simulink model "ES247A_MotAgCmp"  (R2013b)
settings: Solver=VariableStepDiscrete  SolverMode=SingleTasking  StartTime=0.0  StopTime=1  FixedStep=0.002  RelTol=1e-3
values from neighbouring files (symbols this model uses):
  MOTAGCMPENAMASK_CNT_U08 = DataDict.Constant    [ES247A_MotAgCmp_DataDict.m]
  MOTAGCMPMECLDEGPERREV_DEGPERREV_U16P0 = DataDict.Constant    [ES247A_MotAgCmp_DataDict.m]
  MOTAGCUMVALGNDMASK_CNT_U32 = DataDict.Constant    [ES247A_MotAgCmp_DataDict.m]
  MOTAGCUMVALGNDMRFREVMASK_CNT_U32 = DataDict.Constant    [ES247A_MotAgCmp_DataDict.m]
  MOTAGDELTALIM_MOTREV_U0P16 = DataDict.Constant    [ES247A_MotAgCmp_DataDict.m]
  MOTAGMAXDELTA_MOTREV_U0P16 = DataDict.Constant    [ES247A_MotAgCmp_DataDict.m]
  SysGlbPrmMotPoleCnt = DataDict.ImprtdCal    [ES247A_MotAgCmp_DataDict.m]
  SysGlbPrmSysKineRat = DataDict.ImprtdCal    [ES247A_MotAgCmp_DataDict.m]
undefined symbols (not defined in the file or in its folder): sigbuilder_block
libraries: simulink x8, NexteerUtilities x4, FixdToFloat x1
(part 1 of 2)
settings Model: Creator=pz79n7  LastModifiedBy=tzbsjd
settings SolverCC: AutoInsertRateTranBlk=on  InsertRTBMode=Always
settings DataIOCC: LimitDataPoints=off  SaveFormat=Structure  ReturnWorkspaceOutputs=on
settings OptimizationCC: BlockReduction=off  InlineParams=on  ZeroExternalMemoryAtStartup=off  ZeroInternalMemoryAtStartup=off  OptimizeModelRefInitCode=on  LifeSpan=1
settings DebuggingCC: SignalInfNanChecking=error  SignalRangeChecking=warning  UnderspecifiedInitializationDetection=Simplified  SolverPrmCheckMsg=error  InheritedTsInSrcMsg=error  DiscreteInheritContinuousMsg=error  SingleTaskRateTransMsg=error  TasksWithSamePriorityMsg=error  SigSpecEnsureSampleTimeMsg=error  CheckMatrixSingularityMsg=error  ParameterUnderflowMsg=error  ParameterPrecisionLossMsg=error  ParameterTunabilityLossMsg=error  FixptConstUnderflowMsg=warning  FixptConstOverflowMsg=warning  VectorMatrixConversionMsg=error  SignalLabelMismatchMsg=error  UnconnectedInputMsg=error  UnconnectedOutputMsg=error  UnconnectedLineMsg=error  SFcnCompatibilityMsg=error  UniqueDataStoreMsg=warning  BusObjectLabelMismatch=error  RootOutportRequireBusObject=error  AssertControl=DisableAll  ModelReferenceIOMsg=error  ModelReferenceVersionMismatchMessage=warning  ModelReferenceIOMismatchMessage=error  ModelReferenceCSMismatchMessage=warning  ModelReferenceDataLoggingMessage=error  StateNameClashWarn=warning  StrictBusMsg=ErrorOnBusTreatedAsVector  NonBusSignalsTreatedAsBus=error  SFUnexpectedBacktrackingDiag=error  SFInvalidInputDataAccessInChartInitDiag=error  SFNoUnconditionalDefaultTransitionDiag=error  SFTransitionOutsideNaturalParentDiag=error  SFUnconditionalTransitionShadowingDiag=error  SFUndirectedBroadcastEventsDiag=error
settings ModelReferenceCC: ModelReferenceNumInstancesAllowed=Single
settings RTWCC: SystemTargetFile=autosar.tlc  GenCodeOnly=on  TemplateMakefile=ert_default_tmf  Description=AUTOSAR  GenerateReport=on  ProcessScript=autosar_make_rtw_hook  LaunchReport=on
settings CodeAppCC: GenerateComments=off  IgnoreCustomStorageClasses=off  CustomSymbolStrType=$N$R$M  CustomSymbolStrBlkIO=$N$M  SimulinkBlockComments=off
settings STFCustomTargetCC: ParMdlRefBuildCompliant=on  CompOptLevelCompliant=on  IncludeMdlTerminateFcn=off  CombineOutputUpdateFcns=on  SuppressErrorStatus=on  ERTFirstTimeCompliant=on  ERTCustomFileBanners=on  SupportNonFinite=off  SupportComplex=off  SupportContinuousTime=off  SupportNonInlinedSFcns=off  MATLABClassNameForMDSCustomization=Simulink.SoftwareTarget.ERTCustomization  AutosarCompliant=on  GRTInterface=off  SystemTargetFile=autosar.tlc
settings ERTTargetCC: CodeReplacementLibrary=ANSI_C  ConcurrentExecutionCompliant=off  IncludeMdlTerminateFcn=off  SuppressErrorStatus=on  SupportNonFinite=off  SupportComplex=off  ModelStepFunctionPrototypeControlCompliant=off  CPPClassGenCompliant=off  AutosarCompliant=on  InlinedParameterPlacement=NonHierarchical  ERTCustomFileTemplate=example_file_process.tlc  EnableUserReplacementTypes=on

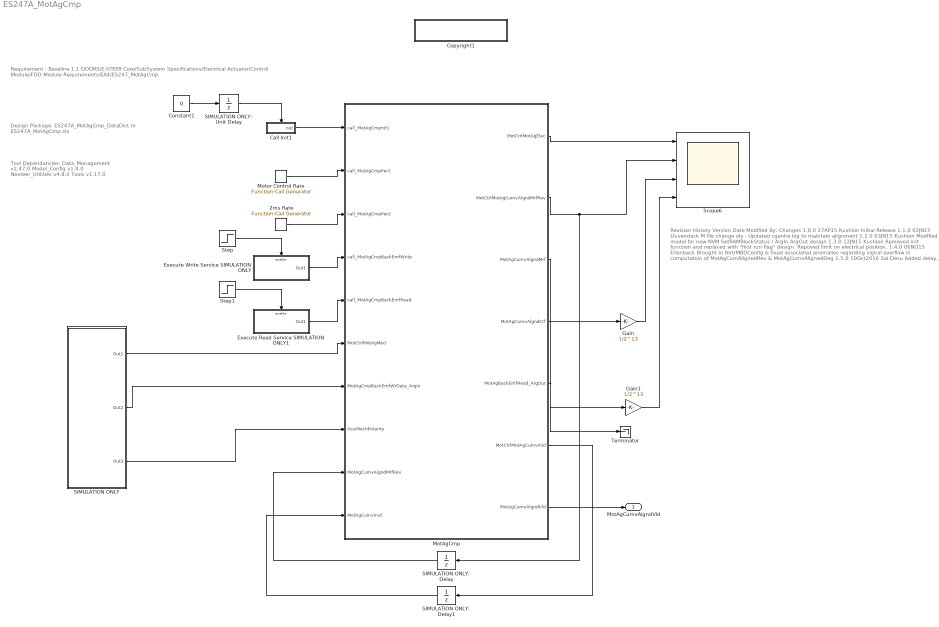
== system ES247A_MotAgCmp ==
  note: Revision History
      |
      | Version		Date 		Modified By: 		Changes
      | 1.0.0	 	27AP15		Kushion			Initial Release
      | 1.1.0		02JN15		Duvendack		M file change oly - Updated cganhe log to maintain alignment
      | 1.2.0		03JN15		Kushion			Modified model for new NVM SetRAMBlockStatus / ArgIn ArgOut design
      | 1.3.0		12JN15		Kushion			Removed init function and replaced with "first run flag" design.  Repoved limit on electrical position.
      | 1.4.0		06NO15		Erlenbeck		Brought in NxtrMBDConfig & fixed associated anomalies regarding signal overflow in computatoin
      | 										of MotAgCumAlignedRev & MotAgCumvAlignedDeg
      | 1.5.0              10Oct2016     Sai Desu              Added delay to use MotCntrlMotAgMecl
      | 1.6.0              19Oct2016     Sai Desu             Moved MotAgCmpMotCtrlMotAgMeclPrev store to outside of the subsystem
      | 1.7.0               11Nov2016    Sai Desu             Added a new PIM DigMotHwPosn for EMC Validation
  note: Tool Dependancies:
      | Data_Management v2.47.0
      | Model_Config v1.4.0
      | Nexteer_Utilities v4.8.0
      | Tools v1.17.0
  note: Requirement : Baseline 1.1
      | DOORS/E-STEER Core/SubSystem Specifications/Electrical Actuator/Control Module/FDD Module Requirements/EA4/ES247_MotAgCmp
  note: Design Package:
      | ES247A_MotAgCmp_DataDict.m
      | ES247A_MotAgCmp.slx
  2ms Rate : simulink/Ports & Subsystems/Function-Call Generator  sample_time=0.002  numberOfIterations=1
  Call Init1 : Subsystem  TreatAsAtomicUnit=on
  Constant1 : Constant  Value=0  OutDataTypeStr=uint8
  Copyright1 : Subsystem  Description=|  mask(Copyright Information){none=on}
      | Copyright info block.                                               
      |                                                                     
      | Place copyright information at the top of every subsystem in design.
      mask prompts: none "No parameters"
      mask help: Place copyright information at the top of every subsystem in design.
      mask Display:
      | NxtrConf = 'Nexteer Confidential';
      | 
      | sys = bdroot; %handle for the current model ("system")
      | first = get_param(sys,'Created');
      | if(isempty(first))
      |     first = datestr(now,'yyyy');
      | else
      |     first = first(end-3:end);  %year is last four digits
      | end
      | 
      | last = get_param(sys,'LastModifiedDate');
      | if isempty(last)
      |     last = datestr(now,'yyyy');
      | else
      |     last = last(end-3:end);
      | end
      | 
      | if strcmp(first,last)
      |     fprintf('%s\nCopyright  %s Nexteer',NxtrConf,first);
      | else
      |     fprintf('%s\n%s%s-%s Nexteer',NxtrConf,char(169),first,last);
      | end
  Execute Read Service SIMULATION ONLY1 : Subsystem  TreatAsAtomicUnit=on
  Execute Write Service SIMULATION ONLY : Subsystem  TreatAsAtomicUnit=on
  Gain : Gain  Gain=1/2^13
  Gain1 : Gain  Gain=1/2^13
  MotAgCmp : Subsystem
  Motor Control Rate : simulink/Ports & Subsystems/Function-Call Generator  sample_time=0.0000625  numberOfIterations=1
  SIMULATION ONLY : Subsystem
  SIMULATION ONLY: Delay : UnitDelay  SampleTime=-1
  SIMULATION ONLY: Delay1 : UnitDelay  SampleTime=-1
  SIMULATION ONLY: Unit Delay : UnitDelay  InitialCondition=1  SampleTime=-1
  Scope6 : Scope  NumInputPorts=4
      settings: YMin=0~-1e+08~-200000~-200000  YMax=70000~1.1e+09~200000~200000  SaveName=ScopeData5  MaxDataPoints=100000
  Step : Step  Time=4.175  SampleTime=0
  Step1 : Step  Time=4.185  SampleTime=0
  Terminator : Terminator
  MotAgCumvAlgndVld : Outport  RequirementInfo={} %GIDa_42b80226_dd05_44ce_a302_5ea1a8b1de89
  wires:
  MotAgCmp/1(MotCtrlMotAgElec) -> Scope6/1
  MotAgCmp/2(MotCtrlMotAgCumvAlgndMrfRev) -> SIMULATION ONLY: Delay/1, Scope6/2
  Motor Control Rate/1 -> MotAgCmp/2(call_MotAgCmpPer1)
  Execute Write Service SIMULATION ONLY/1(Out1) -> MotAgCmp/4(call_MotAgCmpBackEmfWrite)
  Step/1 -> Execute Write Service SIMULATION ONLY/Enable
  2ms Rate/1 -> MotAgCmp/3(call_MotAgCmpPer2)
  MotAgCmp/3(MotAgCumvAlgndMrf) -> Gain/1
  MotAgCmp/4(MotAgCumvAlgndCrf) -> Gain1/1
  SIMULATION ONLY/3(Out3) -> MotAgCmp/8(AssiMechPolarity)
  SIMULATION ONLY/1(Out1) -> MotAgCmp/6(MotCtrlMotAgMecl)
  SIMULATION ONLY/2(Out2) -> MotAgCmp/7(MotAgCmpBackEmfWrData_ArgIn)
  Execute Read Service SIMULATION ONLY1/1(Out1) -> MotAgCmp/5(call_MotAgCmpBackEmfRead)
  Step1/1 -> Execute Read Service SIMULATION ONLY1/Enable
  Gain/1 -> Scope6/3
  Gain1/1 -> Scope6/4
  MotAgCmp/5(MotAgBackEmfRead_ArgOut) -> Terminator/1
  SIMULATION ONLY: Delay/1 -> MotAgCmp/9(MotAgCumvAlgndMrfRev)
  MotAgCmp/6(MotCtrlMotAgCumvInid) -> SIMULATION ONLY: Delay1/1
  Constant1/1 -> SIMULATION ONLY: Unit Delay/1
  SIMULATION ONLY: Unit Delay/1 -> Call Init1/Enable
  Call Init1/1(out) -> MotAgCmp/1(call_MotAgCmpnit1)
  SIMULATION ONLY: Delay1/1 -> MotAgCmp/10(MotAgCumvInid)
  MotAgCmp/7(MotAgCumvAlgndVld) -> MotAgCumvAlgndVld/1

== system ES247A_MotAgCmp/Call Init1 ==
  Enable : EnablePort
  Function Call Trigger : simulink/Ports & Subsystems/Function-Call Generator  RequirementInfo={} %GIDa_a6a4a62e_0f67_4a31_8bd8_36e712ec7718  sample_time=0.002  numberOfIterations=1
  out : Outport
  wires:
  Function Call Trigger/1 -> out/1

== system ES247A_MotAgCmp/Copyright1 ==

== system ES247A_MotAgCmp/Execute Read Service SIMULATION ONLY1 ==
  Enable : EnablePort
  Function-Call Generator1 : simulink/Ports & Subsystems/Function-Call Generator  sample_time=0.0000625  numberOfIterations=1
  Out1 : Outport
  wires:
  Function-Call Generator1/1 -> Out1/1

== system ES247A_MotAgCmp/Execute Write Service SIMULATION ONLY ==
  Enable : EnablePort
  Function-Call Generator1 : simulink/Ports & Subsystems/Function-Call Generator  sample_time=0.0000625  numberOfIterations=1
  Out1 : Outport
  wires:
  Function-Call Generator1/1 -> Out1/1

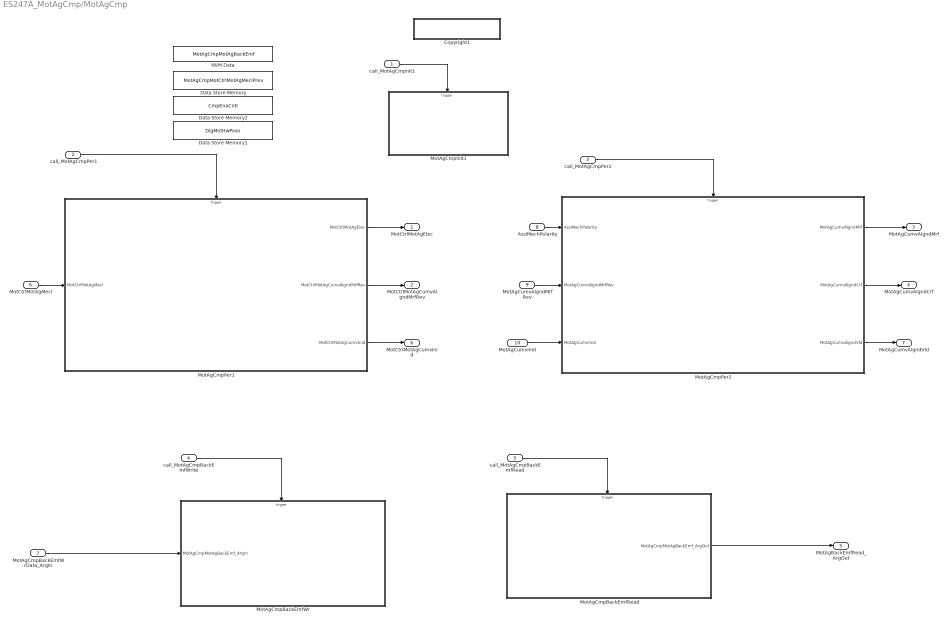
== system ES247A_MotAgCmp/MotAgCmp ==
  call_MotAgCmpnit1 : Inport  RequirementInfo={} %GIDa_7be01678_764c_45c5_827a_c2415c53d3c3
  call_MotAgCmpPer1 : Inport  RequirementInfo={'linktype_rmi_doors' '0000cf60 (/E-STEER Core/SubSystem Specifications/Electrical Actuator/Control Module/FDD Module Requirements/EA4/ES247A_MotAgCmp DRAFT)' '#ES247A_75' 'true' 'REQ: ES247A_75' '' } %GIDa_c4a7fd40_4a5d_4f59_ada5_16c56c4fb6c4  Port=2
  call_MotAgCmpPer2 : Inport  RequirementInfo={} %GIDa_2d6987ea_2640_46d5_a436_3696734fd2e8  Port=3
  call_MotAgCmpBackEmfWrite : Inport  Port=4
  call_MotAgCmpBackEmfRead : Inport  Port=5
  MotCtrlMotAgMecl : Inport  RequirementInfo={'linktype_rmi_doors' '0000cf60 (/E-STEER Core/SubSystem Specifications/Electrical Actuator/Control Module/FDD Module Requirements/EA4/ES247A_MotAgCmp DRAFT)' '#ES247A_48' 'true' 'REQ: ES247A_48' '' } %GIDa_c8a552f0_582e_4578_bd53_0d3cc336a1f5  Port=6
  MotAgCmpBackEmfWrData_ArgIn : Inport  Port=7
  AssiMechPolarity : Inport  RequirementInfo={'linktype_rmi_doors' '0000cf60 (/E-STEER Core/SubSystem Specifications/Electrical Actuator/Control Module/FDD Module Requirements/EA4/ES247A_MotAgCmp DRAFT)' '#ES247A_49' 'true' 'REQ: ES247A_49' '' } %GIDa_2804f92e_c79f_4452_aaac_51e06974467c  Port=8
  MotAgCumvAlgndMrfRev : Inport  RequirementInfo={'linktype_rmi_doors' '0000cf60 (/E-STEER Core/SubSystem Specifications/Electrical Actuator/Control Module/FDD Module Requirements/EA4/ES247A_MotAgCmp DRAFT)' '#ES247A_49' 'true' 'REQ: ES247A_49' '' } %GIDa_aef0170f_c17e_4400_b85e_a6e7f6d587e0  Port=9
  MotAgCumvInid : Inport  Port=10
  Copyright1 : Subsystem  Description=|  mask(Copyright Information){none=on}
      | Copyright info block.                                               
      |                                                                     
      | Place copyright information at the top of every subsystem in design.
      mask prompts: none "No parameters"
      mask help: Place copyright information at the top of every subsystem in design.
      mask Display:
      | NxtrConf = 'Nexteer Confidential';
      | 
      | sys = bdroot; %handle for the current model ("system")
      | first = get_param(sys,'Created');
      | if(isempty(first))
      |     first = datestr(now,'yyyy');
      | else
      |     first = first(end-3:end);  %year is last four digits
      | end
      | 
      | last = get_param(sys,'LastModifiedDate');
      | if isempty(last)
      |     last = datestr(now,'yyyy');
      | else
      |     last = last(end-3:end);
      | end
      | 
      | if strcmp(first,last)
      |     fprintf('%s\nCopyright  %s Nexteer',NxtrConf,first);
      | else
      |     fprintf('%s\n%s%s-%s Nexteer',NxtrConf,char(169),first,last);
      | end
  Data Store Memory : DataStoreMemory  DataStoreName=MotAgCmpMotCtrlMotAgMeclPrev  StateMustResolveToSignalObject=on
  Data Store Memory1 : DataStoreMemory  DataStoreName=DigMotHwPosn  OutDataTypeStr=single  StateMustResolveToSignalObject=on
  Data Store Memory2 : DataStoreMemory  DataStoreName=CmpEnaCntr  OutDataTypeStr=uint8  StateMustResolveToSignalObject=on
  MotAgCmpBackEmfRead : Subsystem  RequirementInfo={'linktype_rmi_doors' '0000cf60 (/E-STEER Core/SubSystem Specifications/Electrical Actuator/Control Module/FDD Module Requirements/EA4/ES247A_MotAgCmp DRAFT)' '#ES247A_71' 'true' 'REQ: ES247A_71' '' } %GIDa_3ab88c9c_8789_4b0d_9902_4656dd01c1af
  MotAgCmpBackEmfWr : Subsystem  RequirementInfo={'linktype_rmi_doors' '0000cf60 (/E-STEER Core/SubSystem Specifications/Electrical Actuator/Control Module/FDD Module Requirements/EA4/ES247A_MotAgCmp DRAFT)' '#ES247A_32' 'true' 'REQ: ES247A_32' '' } %GIDa_04a0761c_e8f1_4ec8_a62e_de9528ead8f5
  MotAgCmpInit1 : Subsystem
  MotAgCmpPer1 : Subsystem
  MotAgCmpPer2 : Subsystem  RequirementInfo={'linktype_rmi_doors' '0000cf60 (/E-STEER Core/SubSystem Specifications/Electrical Actuator/Control Module/FDD Module Requirements/EA4/ES247A_MotAgCmp DRAFT)' '#ES247A_81' 'true' 'REQ: ES247A_81' '' ; 'linktype_rmi_doors' '0000cf60 (/E-STEER Core/SubSystem Specifications/Electrical Actuator/Control Module/FDD Module Requirements/EA4/ES247A_MotAgCmp)' '#ES247A_82' 'true' 'REQ: ES247A_82' '' } %GIDa_e65ac8e8_9ab9_42a4_b83b_13d5ab48a7a2
  NVM Data : DataStoreMemory  DataStoreName=MotAgCmpMotAgBackEmf  StateMustResolveToSignalObject=on
  MotCtrlMotAgElec : Outport  RequirementInfo={'linktype_rmi_doors' '0000cf60 (/E-STEER Core/SubSystem Specifications/Electrical Actuator/Control Module/FDD Module Requirements/EA4/ES247A_MotAgCmp DRAFT)' '#ES247A_51' 'true' 'REQ: ES247A_51' '' } %GIDa_6b71c28c_c263_4ab9_a9ff_dc75eb086ef7
  MotCtrlMotAgCumvAlgndMrfRev : Outport  RequirementInfo={'linktype_rmi_doors' '0000cf60 (/E-STEER Core/SubSystem Specifications/Electrical Actuator/Control Module/FDD Module Requirements/EA4/ES247A_MotAgCmp DRAFT)' '#ES247A_52' 'true' 'REQ: ES247A_52' '' } %GIDa_7f7a1133_6478_44cc_ba52_f9cd2e5fc496  Port=2
  MotAgCumvAlgndMrf : Outport  RequirementInfo={'linktype_rmi_doors' '0000cf60 (/E-STEER Core/SubSystem Specifications/Electrical Actuator/Control Module/FDD Module Requirements/EA4/ES247A_MotAgCmp DRAFT)' '#ES247A_65' 'true' 'REQ: ES247A_65' '' } %GIDa_e8cf59a5_0afd_4c9b_ac68_3f78ef6fc2e1  Port=3
  MotAgCumvAlgndCrf : Outport  RequirementInfo={'linktype_rmi_doors' '0000cf60 (/E-STEER Core/SubSystem Specifications/Electrical Actuator/Control Module/FDD Module Requirements/EA4/ES247A_MotAgCmp DRAFT)' '#ES247A_66' 'true' 'REQ: ES247A_66' '' } %GIDa_3d536a6e_6a87_451d_a4a3_e4fd4989ea47  Port=4
  MotAgBackEmfRead_ArgOut : Outport  Port=5
  MotCtrlMotAgCumvInid : Outport  RequirementInfo={} %GIDa_86bc0d61_8c02_41ab_9ce1_f07b2e2a042f  Port=6
  MotAgCumvAlgndVld : Outport  RequirementInfo={} %GIDa_abce87f6_0981_4822_b74c_d0d31c59bc53  Port=7
  wires:
  MotCtrlMotAgMecl/1 -> MotAgCmpPer1/1(MotCtrlMotAgMecl)
  call_MotAgCmpPer1/1 -> MotAgCmpPer1/Trigger
  call_MotAgCmpBackEmfWrite/1 -> MotAgCmpBackEmfWr/Trigger
  MotAgCmpPer1/2(MotCtrlMotAgCumvAlgndMrfRev) -> MotCtrlMotAgCumvAlgndMrfRev/1
  AssiMechPolarity/1 -> MotAgCmpPer2/1(AssiMechPolarity)
  call_MotAgCmpPer2/1 -> MotAgCmpPer2/Trigger
  call_MotAgCmpBackEmfRead/1 -> MotAgCmpBackEmfRead/Trigger
  MotAgCmpBackEmfRead/1(MotAgCmpMotAgBackEmf_ArgOut) -> MotAgBackEmfRead_ArgOut/1
  MotAgCmpPer1/1(MotCtrlMotAgElec) -> MotCtrlMotAgElec/1
  MotAgCmpPer2/1(MotAgCumvAlgndMrf) -> MotAgCumvAlgndMrf/1
  MotAgCmpPer2/2(MotAgCumvAlgndCrf) -> MotAgCumvAlgndCrf/1
  MotAgCmpBackEmfWrData_ArgIn/1 -> MotAgCmpBackEmfWr/1(MotAgCmpMotAgBackEmf_ArgIn)
  MotAgCumvAlgndMrfRev/1 -> MotAgCmpPer2/2(MotAgCumvAlgndMrfRev)
  MotAgCmpPer1/3(MotCtrlMotAgCumvInid) -> MotCtrlMotAgCumvInid/1
  call_MotAgCmpnit1/1 -> MotAgCmpInit1/Trigger
  MotAgCumvInid/1 -> MotAgCmpPer2/3(MotAgCumvInid)
  MotAgCmpPer2/3(MotAgCumvAlgndVld) -> MotAgCumvAlgndVld/1

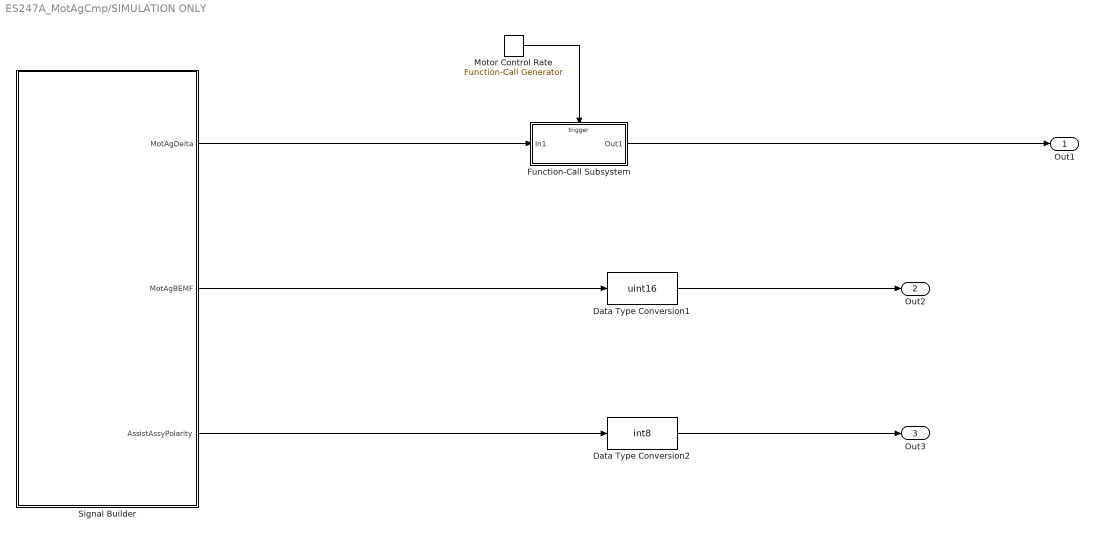
== system ES247A_MotAgCmp/SIMULATION ONLY ==
  Data Type Conversion1 : DataTypeConversion  OutDataTypeStr=uint16  RndMeth=Nearest
  Data Type Conversion2 : DataTypeConversion  OutDataTypeStr=int8  RndMeth=Nearest
  Function-Call Subsystem : Subsystem  TreatAsAtomicUnit=on
  Motor Control Rate : simulink/Ports & Subsystems/Function-Call Generator  sample_time=0.005  numberOfIterations=1
  Signal Builder : Subsystem  Tag=STV Subsys  LoadFcn=sigbuilder_block('load');  StartFcn=sigbuilder_block('start');  StopFcn=sigbuilder_block('stop');  ClipboardFcn=sigbuilder_block('clipboard');  mask(Sigbuilder block){}
      mask help: Simulink:masks:SigbuilderBlock_MD
      mask init:
      | if ~strcmp(get_param(bdroot(gcbh),'SimulationStatus'),'stopped') tuvar = sigbuilder_block('maskInit'); end
      settings: CopyFcn=sigbuilder_block('copy');  DeleteFcn=sigbuilder_block('delete');  ModelCloseFcn=sigbuilder_block('modelClose');  PreSaveFcn=sigbuilder_block('preSave');  PauseFcn=sigbuilder_block('pause');  ContinueFcn=sigbuilder_block('continue');  NameChangeFcn=sigbuilder_block('namechange');  OpenFcn=sigbuilder_block('open',[65.25 264.75 1018.5 480.75 ]);  CloseFcn=sigbuilder_block('close');
      mask Display: plot(0, 0, 100, 100,[2, 2, 32, 32, 2], [68, 8, 8, 68, 68],[32, 2], [38, 38], [32, 19, 2],[53, 60, 44], [32, 17, 17, 2],[16, 16, 31, 31]);txt = getActiveGroup(gcbh);text(2, 100, txt,'verticalAlignment', 'top');
  Out1 : Outport
  Out2 : Outport  Port=2
  Out3 : Outport  Port=3
  wires:
  Signal Builder/2(MotAgBEMF) -> Data Type Conversion1/1
  Signal Builder/3(AssistAssyPolarity) -> Data Type Conversion2/1
  Signal Builder/1(MotAgDelta) -> Function-Call Subsystem/1(In1)
  Data Type Conversion1/1 -> Out2/1
  Data Type Conversion2/1 -> Out3/1
  Motor Control Rate/1 -> Function-Call Subsystem/Trigger
  Function-Call Subsystem/1(Out1) -> Out1/1

== system ES247A_MotAgCmp/MotAgCmp/Copyright1 ==

== system ES247A_MotAgCmp/MotAgCmp/MotAgCmpBackEmfRead ==
  Trigger : TriggerPort  TriggerType=function-call  PortDimensions=1
  Copyright1 : Subsystem  Description=|  mask(Copyright Information){none=on}
      | Copyright info block.                                               
      |                                                                     
      | Place copyright information at the top of every subsystem in design.
      mask prompts: none "No parameters"
      mask help: Place copyright information at the top of every subsystem in design.
      mask Display:
      | NxtrConf = 'Nexteer Confidential';
      | 
      | sys = bdroot; %handle for the current model ("system")
      | first = get_param(sys,'Created');
      | if(isempty(first))
      |     first = datestr(now,'yyyy');
      | else
      |     first = first(end-3:end);  %year is last four digits
      | end
      | 
      | last = get_param(sys,'LastModifiedDate');
      | if isempty(last)
      |     last = datestr(now,'yyyy');
      | else
      |     last = last(end-3:end);
      | end
      | 
      | if strcmp(first,last)
      |     fprintf('%s\nCopyright  %s Nexteer',NxtrConf,first);
      | else
      |     fprintf('%s\n%s%s-%s Nexteer',NxtrConf,char(169),first,last);
      | end
  Data Store Read : DataStoreRead  DataStoreName=MotAgCmpMotAgBackEmf
  MotAgCmpMotAgBackEmf_ArgOut : Outport
  wires:
  Data Store Read/1 -> MotAgCmpMotAgBackEmf_ArgOut/1  "MotAgCmpMotAgBackEmf_ArgOut"

== system ES247A_MotAgCmp/MotAgCmp/MotAgCmpBackEmfWr ==
  MotAgCmpMotAgBackEmf_ArgIn : Inport
  Trigger : TriggerPort  TriggerType=function-call  PortDimensions=1
  Constant : Constant
  Copyright1 : Subsystem  Description=|  mask(Copyright Information){none=on}
      | Copyright info block.                                               
      |                                                                     
      | Place copyright information at the top of every subsystem in design.
      mask prompts: none "No parameters"
      mask help: Place copyright information at the top of every subsystem in design.
      mask Display:
      | NxtrConf = 'Nexteer Confidential';
      | 
      | sys = bdroot; %handle for the current model ("system")
      | first = get_param(sys,'Created');
      | if(isempty(first))
      |     first = datestr(now,'yyyy');
      | else
      |     first = first(end-3:end);  %year is last four digits
      | end
      | 
      | last = get_param(sys,'LastModifiedDate');
      | if isempty(last)
      |     last = datestr(now,'yyyy');
      | else
      |     last = last(end-3:end);
      | end
      | 
      | if strcmp(first,last)
      |     fprintf('%s\nCopyright  %s Nexteer',NxtrConf,first);
      | else
      |     fprintf('%s\n%s%s-%s Nexteer',NxtrConf,char(169),first,last);
      | end
  Data Store Write : DataStoreWrite  DataStoreName=MotAgCmpMotAgBackEmf
  MotAgCmpMotAgBackEmf_SetRamBlockStatus : Subsystem
  wires:
  MotAgCmpMotAgBackEmf_ArgIn/1 -> Data Store Write/1
  Constant/1 -> MotAgCmpMotAgBackEmf_SetRamBlockStatus/1(BlockChanged)

== system ES247A_MotAgCmp/MotAgCmp/MotAgCmpInit1 ==
  note: Do Nothing
  function : TriggerPort  TriggerType=function-call
  CopyRight2 : Subsystem  Description=|  mask(Copyright Information){none=on}
      | Copyright info block.                                               
      |                                                                     
      | Place copyright information at the top of every subsystem in design.
      mask prompts: none "No parameters"
      mask help: Place copyright information at the top of every subsystem in design.
      mask Display:
      | NxtrConf = 'Nexteer Confidential';
      | 
      | sys = bdroot; %handle for the current model ("system")
      | first = get_param(sys,'Created');
      | first = first(end-3:end);  %year is last four digits
      | 
      | last = get_param(sys,'LastModifiedDate');
      | if isempty(last)
      |     last = datestr(now,'yyyy');
      | else
      |     last = last(end-3:end);
      | end
      | 
      | if strcmp(first,last)
      |     fprintf('%s -- Copyright %s Nexteer',NxtrConf,first)
      | else
      |     fprintf('%s -- %s%s- %s Nexteer',NxtrConf,char(169),first,last)
      | end

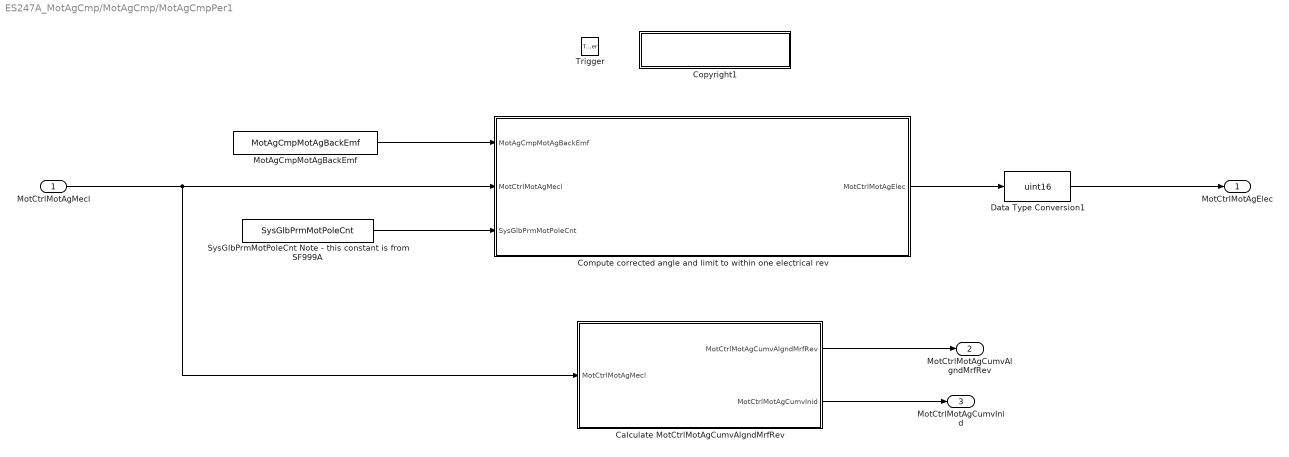
== system ES247A_MotAgCmp/MotAgCmp/MotAgCmpPer1 ==
  MotCtrlMotAgMecl : Inport
  Trigger : TriggerPort  TriggerType=function-call  PortDimensions=1
  Calculate MotCtrlMotAgCumvAlgndMrfRev : Subsystem  RequirementInfo={'linktype_rmi_doors' '0000cf60 (/E-STEER Core/SubSystem Specifications/Electrical Actuator/Control Module/FDD Module Requirements/EA4/ES247A_MotAgCmp)' '#ES247A_80' 'true' 'REQ: ES247A_80' '' ; 'linktype_rmi_doors' '0000cf60 (/E-STEER Core/SubSystem Specifications/Electrical Actuator/Control Module/FDD Module Requirements/EA4/ES247A_MotAgCmp)' '#ES247A_69' 'true' 'REQ: ES247A_69' '' } %GIDa_5bbbb2b0_d947_418a_8c61_c0f17c4aa380  TreatAsAtomicUnit=on
  Compute corrected angle and limit to within one electrical rev : Stateflow chart  RequirementInfo={'linktype_rmi_doors' '0000cf60 (/E-STEER Core/SubSystem Specifications/Electrical Actuator/Control Module/FDD Module Requirements/EA4/ES247A_MotAgCmp DRAFT)' '#ES247A_83' 'true' 'REQ: ES247A_83' '' ; 'linktype_rmi_doors' '0000cf60 (/E-STEER Core/SubSystem Specifications/Electrical Actuator/Control Module/FDD Module Requirements/EA4/ES247A_MotAgCmp DRAFT)' '#ES247A_67' 'true' 'REQ: ES247A_67' '' } %GIDa_5a42319c_60b6_4e66_9128_72202dd936e3  TreatAsAtomicUnit=on
  Copyright1 : Subsystem  Description=|  mask(Copyright Information){none=on}
      | Copyright info block.                                               
      |                                                                     
      | Place copyright information at the top of every subsystem in design.
      mask prompts: none "No parameters"
      mask help: Place copyright information at the top of every subsystem in design.
      mask Display:
      | NxtrConf = 'Nexteer Confidential';
      | 
      | sys = bdroot; %handle for the current model ("system")
      | first = get_param(sys,'Created');
      | if(isempty(first))
      |     first = datestr(now,'yyyy');
      | else
      |     first = first(end-3:end);  %year is last four digits
      | end
      | 
      | last = get_param(sys,'LastModifiedDate');
      | if isempty(last)
      |     last = datestr(now,'yyyy');
      | else
      |     last = last(end-3:end);
      | end
      | 
      | if strcmp(first,last)
      |     fprintf('%s\nCopyright  %s Nexteer',NxtrConf,first);
      | else
      |     fprintf('%s\n%s%s-%s Nexteer',NxtrConf,char(169),first,last);
      | end
  Data Type Conversion1 : DataTypeConversion  RequirementInfo={'linktype_rmi_doors' '0000cf60 (/E-STEER Core/SubSystem Specifications/Electrical Actuator/Control Module/FDD Module Requirements/EA4/ES247A_MotAgCmp DRAFT)' '#ES247A_67' 'true' 'REQ: ES247A_67' '' } %GIDa_26f4a4f6_3ed1_4b92_8cf7_4163e6d2cb61  OutDataTypeStr=uint16
  MotAgCmpMotAgBackEmf : DataStoreRead  RequirementInfo={'linktype_rmi_doors' '0000cf60 (/E-STEER Core/SubSystem Specifications/Electrical Actuator/Control Module/FDD Module Requirements/EA4/ES247A_MotAgCmp DRAFT)' '#ES247A_53' 'true' 'REQ: ES247A_53' '' ; 'linktype_rmi_doors' '0000cf60 (/E-STEER Core/SubSystem Specifications/Electrical Actuator/Control Module/FDD Module Requirements/EA4/ES247A_MotAgCmp DRAFT)' '#ES247A_67' 'true' 'REQ: ES247A_67' '' } %GIDa_10329906_ccbb_4157_8353_939c8ee01137  DataStoreName=MotAgCmpMotAgBackEmf
  SysGlbPrmMotPoleCnt Note - this constant is from SF999A : Constant  RequirementInfo={'linktype_rmi_doors' '0000cf60 (/E-STEER Core/SubSystem Specifications/Electrical Actuator/Control Module/FDD Module Requirements/EA4/ES247A_MotAgCmp DRAFT)' '#ES247A_83' 'true' 'REQ: ES247A_83' '' } %GIDa_8e3881c9_6938_45cd_993e_bed16e6ab181  Value=SysGlbPrmMotPoleCnt
  MotCtrlMotAgElec : Outport  RequirementInfo={'linktype_rmi_doors' '0000cf60 (/E-STEER Core/SubSystem Specifications/Electrical Actuator/Control Module/FDD Module Requirements/EA4/ES247A_MotAgCmp DRAFT)' '#ES247A_67' 'true' 'REQ: ES247A_67' '' } %GIDa_cfebbb21_3d4e_4cdc_a747_9faf534dc136
  MotCtrlMotAgCumvAlgndMrfRev : Outport  RequirementInfo={'linktype_rmi_doors' '0000cf60 (/E-STEER Core/SubSystem Specifications/Electrical Actuator/Control Module/FDD Module Requirements/EA4/ES247A_MotAgCmp DRAFT)' '#ES247A_69' 'true' 'REQ: ES247A_69' '' } %GIDa_94b14ff5_c05a_4ac4_8b30_22f14e9712b7  Port=2
  MotCtrlMotAgCumvInid : Outport  RequirementInfo={} %GIDa_34bf7259_46fe_45de_97e0_bf42a6245edb  Port=3
  wires:
  Calculate MotCtrlMotAgCumvAlgndMrfRev/1(MotCtrlMotAgCumvAlgndMrfRev) -> MotCtrlMotAgCumvAlgndMrfRev/1
  Compute corrected angle and limit to within one electrical rev/1(MotCtrlMotAgElec) -> Data Type Conversion1/1
  MotAgCmpMotAgBackEmf/1 -> Compute corrected angle and limit to within one electrical rev/1(MotAgCmpMotAgBackEmf)
  SysGlbPrmMotPoleCnt Note - this constant is from SF999A/1 -> Compute corrected angle and limit to within one electrical rev/3(SysGlbPrmMotPoleCnt)
  Data Type Conversion1/1 -> MotCtrlMotAgElec/1
  MotCtrlMotAgMecl/1 -> Compute corrected angle and limit to within one electrical rev/2(MotCtrlMotAgMecl), Calculate MotCtrlMotAgCumvAlgndMrfRev/1(MotCtrlMotAgMecl)
  Calculate MotCtrlMotAgCumvAlgndMrfRev/2(MotCtrlMotAgCumvInid) -> MotCtrlMotAgCumvInid/1

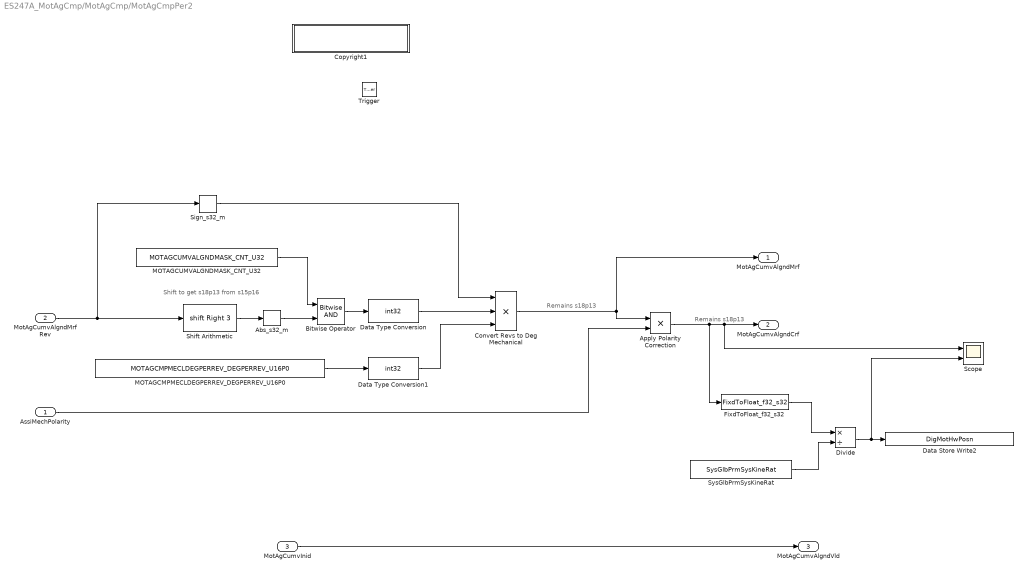
== system ES247A_MotAgCmp/MotAgCmp/MotAgCmpPer2 ==
  note: Shift to get s18p13 from s15p16
  note: Remains s18p13
  note: Remains s18p13
  AssiMechPolarity : Inport
  MotAgCumvAlgndMrfRev : Inport  Port=2
  MotAgCumvInid : Inport  Port=3
  Trigger : TriggerPort  TriggerType=function-call  PortDimensions=1
  Abs_s32_m : NexteerUtilities/Abs_s32_m
      settings: AttributesFormatString=Abs_s32
  "Apply Polarity Correction " : Product  RequirementInfo={'linktype_rmi_doors' '0000cf60 (/E-STEER Core/SubSystem Specifications/Electrical Actuator/Control Module/FDD Module Requirements/EA4/ES247A_MotAgCmp DRAFT)' '#ES247A_82' 'true' 'REQ: ES247A_82' '' } %GIDa_4055bf56_7453_45c2_ba49_95328f4f5f88  OutDataTypeStr=int32
  Bitwise Operator : simulink/Logic and Bit Operations/Bitwise Operator  logicop=AND  UseBitMask=off  NumInputPorts=2  BitMask=bin2dec('11011001')  BitMaskRealWorld=Stored Integer
  Convert Revs to Deg Mechanical : Product  RequirementInfo={'linktype_rmi_doors' '0000cf60 (/E-STEER Core/SubSystem Specifications/Electrical Actuator/Control Module/FDD Module Requirements/EA4/ES247A_MotAgCmp DRAFT)' '#ES247A_81' 'true' 'REQ: ES247A_81' '' } %GIDa_c391b3ab_264a_4521_a26d_e9b9c4e80478  Inputs=3  OutDataTypeStr=int32
  Copyright1 : Subsystem  Description=|  mask(Copyright Information){none=on}
      | Copyright info block.                                               
      |                                                                     
      | Place copyright information at the top of every subsystem in design.
      mask prompts: none "No parameters"
      mask help: Place copyright information at the top of every subsystem in design.
      mask Display:
      | NxtrConf = 'Nexteer Confidential';
      | 
      | sys = bdroot; %handle for the current model ("system")
      | first = get_param(sys,'Created');
      | if(isempty(first))
      |     first = datestr(now,'yyyy');
      | else
      |     first = first(end-3:end);  %year is last four digits
      | end
      | 
      | last = get_param(sys,'LastModifiedDate');
      | if isempty(last)
      |     last = datestr(now,'yyyy');
      | else
      |     last = last(end-3:end);
      | end
      | 
      | if strcmp(first,last)
      |     fprintf('%s\nCopyright  %s Nexteer',NxtrConf,first);
      | else
      |     fprintf('%s\n%s%s-%s Nexteer',NxtrConf,char(169),first,last);
      | end
  Data Store Write2 : DataStoreWrite  DataStoreName=DigMotHwPosn
  Data Type Conversion : DataTypeConversion  OutDataTypeStr=int32
  Data Type Conversion1 : DataTypeConversion  OutDataTypeStr=int32
  Divide : Product  Inputs=*/  OutDataTypeStr=single
  FixdToFloat_f32_s32 : FixdToFloat/FixdToFloat_f32_s32  Param1=13
  MOTAGCMPMECLDEGPERREV_DEGPERREV_U16P0 : Constant  RequirementInfo={'linktype_rmi_doors' '0000cf60 (/E-STEER Core/SubSystem Specifications/Electrical Actuator/Control Module/FDD Module Requirements/EA4/ES247A_MotAgCmp DRAFT)' '#ES247A_81' 'true' 'REQ: ES247A_81' '' } %GIDa_6e914902_d954_41aa_ba16_fd1416dc5d54  Value=MOTAGCMPMECLDEGPERREV_DEGPERREV_U16P0
  MOTAGCUMVALGNDMASK_CNT_U32 : Constant  RequirementInfo={'linktype_rmi_doors' '0000cf60 (/E-STEER Core/SubSystem Specifications/Electrical Actuator/Control Module/FDD Module Requirements/EA4/ES247A_MotAgCmp DRAFT)' '#ES247A_83' 'true' 'REQ: ES247A_83' '' } %GIDa_fa455573_0873_43fa_8814_cfa12256c194  Value=MOTAGCUMVALGNDMASK_CNT_U32  OutDataTypeStr=uint32
  Scope : Scope  NumInputPorts=2
      settings: YMin=-5~-5  YMax=5~5
  Shift Arithmetic : ArithShift  RequirementInfo={'linktype_rmi_doors' '0000cf60 (/E-STEER Core/SubSystem Specifications/Electrical Actuator/Control Module/FDD Module Requirements/EA4/ES247A_MotAgCmp)' '#ES247A_81' 'true' 'REQ: ES247A_81' '' } %GIDa_770f502c_5114_49c6_b819_03d84146a8cc  BitShiftNumber=3  BitShiftDirection=Right
  Sign_s32_m : NexteerUtilities/Sign_s32_m
      settings: AttributesFormatString=Sign_s32
  "SysGlbPrmSysKineRat " : Constant  RequirementInfo={'linktype_rmi_doors' '0000cf60 (/E-STEER Core/SubSystem Specifications/Electrical Actuator/Control Module/FDD Module Requirements/EA4/ES247A_MotAgCmp DRAFT)' '#ES247A_83' 'true' 'REQ: ES247A_83' '' } %GIDa_6fa9465e_844c_42ce_8fb7_0ec1d4a3453d  Value=SysGlbPrmSysKineRat
  MotAgCumvAlgndMrf : Outport  InitialOutput=0
  MotAgCumvAlgndCrf : Outport  Port=2  InitialOutput=0
  MotAgCumvAlgndVld : Outport  RequirementInfo={} %GIDa_006b6504_b9c8_4ac0_8390_3978553d0ea1  Port=3
  wires:
  MotAgCumvAlgndMrfRev/1 -> Sign_s32_m/1, Shift Arithmetic/1
  "Apply Polarity Correction "/1 -> FixdToFloat_f32_s32/1, Scope/1, MotAgCumvAlgndCrf/1
  Convert Revs to Deg Mechanical/1 -> "Apply Polarity Correction "/1, MotAgCumvAlgndMrf/1
  AssiMechPolarity/1 -> "Apply Polarity Correction "/2
  Shift Arithmetic/1 -> Abs_s32_m/1
  Abs_s32_m/1 -> Bitwise Operator/2
  MOTAGCUMVALGNDMASK_CNT_U32/1 -> Bitwise Operator/1
  Sign_s32_m/1 -> Convert Revs to Deg Mechanical/1
  Bitwise Operator/1 -> Data Type Conversion/1
  MOTAGCMPMECLDEGPERREV_DEGPERREV_U16P0/1 -> Data Type Conversion1/1
  Data Type Conversion1/1 -> Convert Revs to Deg Mechanical/3
  Data Type Conversion/1 -> Convert Revs to Deg Mechanical/2
  MotAgCumvInid/1 -> MotAgCumvAlgndVld/1
  FixdToFloat_f32_s32/1 -> Divide/1
  "SysGlbPrmSysKineRat "/1 -> Divide/2
  Divide/1 -> Scope/2, Data Store Write2/1

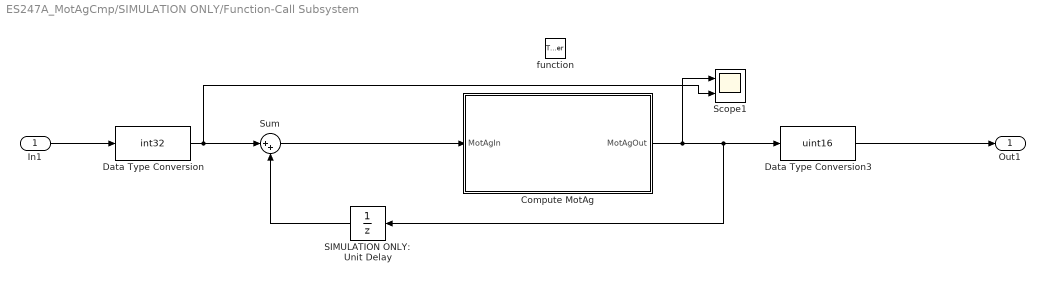
== system ES247A_MotAgCmp/SIMULATION ONLY/Function-Call Subsystem ==
  In1 : Inport
  function : TriggerPort  TriggerType=function-call
  Compute MotAg : Stateflow chart  RequirementInfo={'linktype_rmi_doors' '0000cf60 (/E-STEER Core/SubSystem Specifications/Electrical Actuator/Control Module/FDD Module Requirements/EA4/ES247A_MotAgCmp DRAFT)' '#ES247A_83' 'true' 'REQ: ES247A_83' '' ; 'linktype_rmi_doors' '0000cf60 (/E-STEER Core/SubSystem Specifications/Electrical Actuator/Control Module/FDD Module Requirements/EA4/ES247A_MotAgCmp DRAFT)' '#ES247A_67' 'true' 'REQ: ES247A_67' '' } %GIDa_6496b07e_8496_43fc_b9b6_c819f707934c  TreatAsAtomicUnit=on
  Data Type Conversion : DataTypeConversion  OutDataTypeStr=int32  RndMeth=Nearest
  Data Type Conversion3 : DataTypeConversion  OutDataTypeStr=uint16  RndMeth=Nearest
  SIMULATION ONLY: Unit Delay : UnitDelay  SampleTime=-1
      settings: AttributesFormatString=|
      | InitCond:
      | %<InitialCondition>
  Scope1 : Scope  NumInputPorts=2
      settings: TimeRange=1  YMin=-5~-5  YMax=5~5  SaveName=ScopeData7
  Sum : Sum  Inputs=|++
  Out1 : Outport
  wires:
  Data Type Conversion/1 -> Scope1/2, Sum/1
  SIMULATION ONLY: Unit Delay/1 -> Sum/2
  Compute MotAg/1(MotAgOut) -> Scope1/1, SIMULATION ONLY: Unit Delay/1, Data Type Conversion3/1
  Sum/1 -> Compute MotAg/1(MotAgIn)
  Data Type Conversion3/1 -> Out1/1
  In1/1 -> Data Type Conversion/1

== system ES247A_MotAgCmp/SIMULATION ONLY/Signal Builder ==
  Demux : Demux  Tag=STV Demux  Outputs=3
  FromWs : FromWorkspace  Tag=STV FromWs  VariableName=tuvar  SampleTime=0
      SigBuilderData=|
      | common.afterFinalStr = 'Extrapolate'
      | common.sampleTime = 0
      | dataSet(1).timeRange = [0 1]
      | dataSet(1).name = 'LongRun Overflow'
      | dataSet(2).timeRange = [0 1]
      | dataSet(2).name = 'Group 2'
      | sbobj.Groups(1).Name = 'LongRun Overflow'
      | sbobj.Groups(1).Signals(1).Name = 'MotAgDelta'
      | sbobj.Groups(1).Signals(1).XData = [0 0.009 0.009 0.018 1]
      | sbobj.Groups(1).Signals(1).YData = [1.05 1.05 1.018 1.036 3]
      | sbobj.Groups(1).Signals(2).Name = 'MotAgBEMF'
      | sbobj.Groups(1).Signals(2).XData = [0 1]
      | sbobj.Groups(1).Signals(2).YData = [0 0]
      | sbobj.Groups(1).Signals(3).Name = 'AssistAssyPolarity'
      | sbobj.Groups(1).Signals(3).XData = [0 1]
      | sbobj.Groups(1).Signals(3).YData = [1 1]
      | sbobj.Groups(1).TimeRange = [0 1]
      | sbobj.Groups(2).Name = 'Group 2'
      | sbobj.Groups(2).Signals(1).Name = 'MotAgDelta'
      | sbobj.Groups(2).Signals(1).XData = [0 0.402 0.402 1]
      | sbobj.Groups(2).Signals(1).YData = [4000 4000 -10000 -10000]
      | sbobj.Groups(2).Signals(2).Name = 'MotAgBEMF'
      | sbobj.Groups(2).Signals(2).XData = [0 0.74 0.74 1]
      | sbobj.Groups(2).Signals(2).YData = [0 0 20000 20000]
      | sbobj.Groups(2).Signals(3).Name = 'AssistAssyPolarity'
      | sbobj.Groups(2).Signals(3).XData = [0 0.68 0.68 1]
      | sbobj.Groups(2).Signals(3).YData = [1 1 -1 -1]
      | sbobj.Groups(2).TimeRange = [0 1]
  MotAgDelta : Outport  Tag=STV Outport
  MotAgBEMF : Outport  Tag=STV Outport  Port=2
  AssistAssyPolarity : Outport  Tag=STV Outport  Port=3
  wires:
  Demux/1 -> MotAgDelta/1
  FromWs/1 -> Demux/1
  Demux/2 -> MotAgBEMF/1
  Demux/3 -> AssistAssyPolarity/1

== system ES247A_MotAgCmp/MotAgCmp/MotAgCmpBackEmfRead/Copyright1 ==

== system ES247A_MotAgCmp/MotAgCmp/MotAgCmpBackEmfWr/Copyright1 ==

== system ES247A_MotAgCmp/MotAgCmp/MotAgCmpBackEmfWr/MotAgCmpMotAgBackEmf_SetRamBlockStatus ==
  note: This is the block representing the client call
  BlockChanged : Inport
  Terminator : Terminator
  wires:
  BlockChanged/1 -> Terminator/1

== system ES247A_MotAgCmp/MotAgCmp/MotAgCmpInit1/CopyRight2 ==

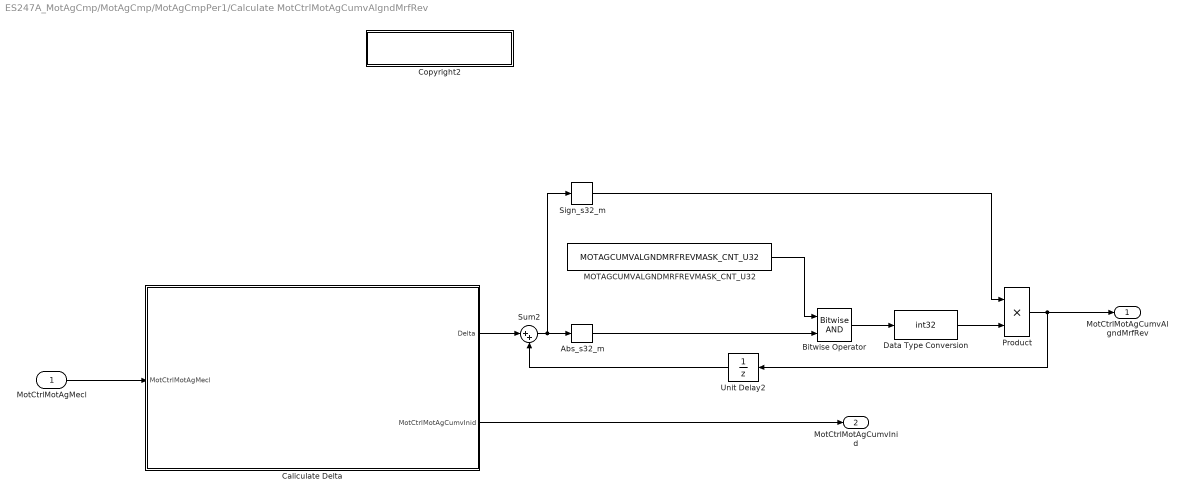
== system ES247A_MotAgCmp/MotAgCmp/MotAgCmpPer1/Calculate MotCtrlMotAgCumvAlgndMrfRev ==
  MotCtrlMotAgMecl : Inport
  Abs_s32_m : NexteerUtilities/Abs_s32_m
      settings: AttributesFormatString=Abs_s32
  Bitwise Operator : simulink/Logic and Bit Operations/Bitwise Operator  logicop=AND  UseBitMask=off  NumInputPorts=2  BitMask=bin2dec('11011001')  BitMaskRealWorld=Stored Integer
  Caliculate Delta : Subsystem
  Copyright2 : Subsystem  Description=|  mask(Copyright Information){none=on}
      | Copyright info block.                                               
      |                                                                     
      | Place copyright information at the top of every subsystem in design.
      mask prompts: none "No parameters"
      mask help: Place copyright information at the top of every subsystem in design.
      mask Display:
      | NxtrConf = 'Nexteer Confidential';
      | 
      | sys = bdroot; %handle for the current model ("system")
      | first = get_param(sys,'Created');
      | if(isempty(first))
      |     first = datestr(now,'yyyy');
      | else
      |     first = first(end-3:end);  %year is last four digits
      | end
      | 
      | last = get_param(sys,'LastModifiedDate');
      | if isempty(last)
      |     last = datestr(now,'yyyy');
      | else
      |     last = last(end-3:end);
      | end
      | 
      | if strcmp(first,last)
      |     fprintf('%s\nCopyright  %s Nexteer',NxtrConf,first);
      | else
      |     fprintf('%s\n%s%s-%s Nexteer',NxtrConf,char(169),first,last);
      | end
  Data Type Conversion : DataTypeConversion  OutDataTypeStr=int32
  MOTAGCUMVALGNDMRFREVMASK_CNT_U32 : Constant  RequirementInfo={'linktype_rmi_doors' '0000cf60 (/E-STEER Core/SubSystem Specifications/Electrical Actuator/Control Module/FDD Module Requirements/EA4/ES247A_MotAgCmp DRAFT)' '#ES247A_83' 'true' 'REQ: ES247A_83' '' } %GIDa_1ac3b4b3_8627_408d_85c8_51492aea6be3  Value=MOTAGCUMVALGNDMRFREVMASK_CNT_U32  OutDataTypeStr=uint32
  Product : Product  RequirementInfo={'linktype_rmi_doors' '0000cf60 (/E-STEER Core/SubSystem Specifications/Electrical Actuator/Control Module/FDD Module Requirements/EA4/ES247A_MotAgCmp DRAFT)' '#ES247A_81' 'true' 'REQ: ES247A_81' '' } %GIDa_494c8fcb_0882_4c39_9df0_c0938aef2f66  OutDataTypeStr=int32
  Sign_s32_m : NexteerUtilities/Sign_s32_m
      settings: AttributesFormatString=Sign_s32
  Sum2 : Sum  RequirementInfo={'linktype_rmi_doors' '0000cf60 (/E-STEER Core/SubSystem Specifications/Electrical Actuator/Control Module/FDD Module Requirements/EA4/ES247A_MotAgCmp DRAFT)' '#ES247A_69' 'true' 'REQ: ES247A_69' '' } %GIDa_7dc143f2_1e32_453c_a88c_7e64883b6643  Inputs=|++  OutDataTypeStr=int32
  Unit Delay2 : UnitDelay  SampleTime=-1  StateName=MotAgCmpMotCtrlMotAgCumvAlgndMrfRevPrev  StateMustResolveToSignalObject=on
      settings: AttributesFormatString=|
      | State Variable:
      | %<StateName>
  MotCtrlMotAgCumvAlgndMrfRev : Outport  RequirementInfo={'linktype_rmi_doors' '0000cf60 (/E-STEER Core/SubSystem Specifications/Electrical Actuator/Control Module/FDD Module Requirements/EA4/ES247A_MotAgCmp DRAFT)' '#ES247A_69' 'true' 'REQ: ES247A_69' '' } %GIDa_72263fd3_04dc_4730_a4ce_e3bb2d637b24
  MotCtrlMotAgCumvInid : Outport  RequirementInfo={} %GIDa_3bd805ae_1a14_41e4_ad0a_9ca54f93dfdb  Port=2
  wires:
  Unit Delay2/1 -> Sum2/2
  Product/1 -> MotCtrlMotAgCumvAlgndMrfRev/1, Unit Delay2/1
  Sum2/1 -> Abs_s32_m/1, Sign_s32_m/1
  Abs_s32_m/1 -> Bitwise Operator/2
  MOTAGCUMVALGNDMRFREVMASK_CNT_U32/1 -> Bitwise Operator/1
  Sign_s32_m/1 -> Product/1
  Bitwise Operator/1 -> Data Type Conversion/1
  Data Type Conversion/1 -> Product/2
  MotCtrlMotAgMecl/1 -> Caliculate Delta/1(MotCtrlMotAgMecl)
  Caliculate Delta/1(Delta) -> Sum2/1
  Caliculate Delta/2(MotCtrlMotAgCumvInid) -> MotCtrlMotAgCumvInid/1

== system ES247A_MotAgCmp/MotAgCmp/MotAgCmpPer1/Copyright1 ==

== system ES247A_MotAgCmp/MotAgCmp/MotAgCmpPer2/Copyright1 ==

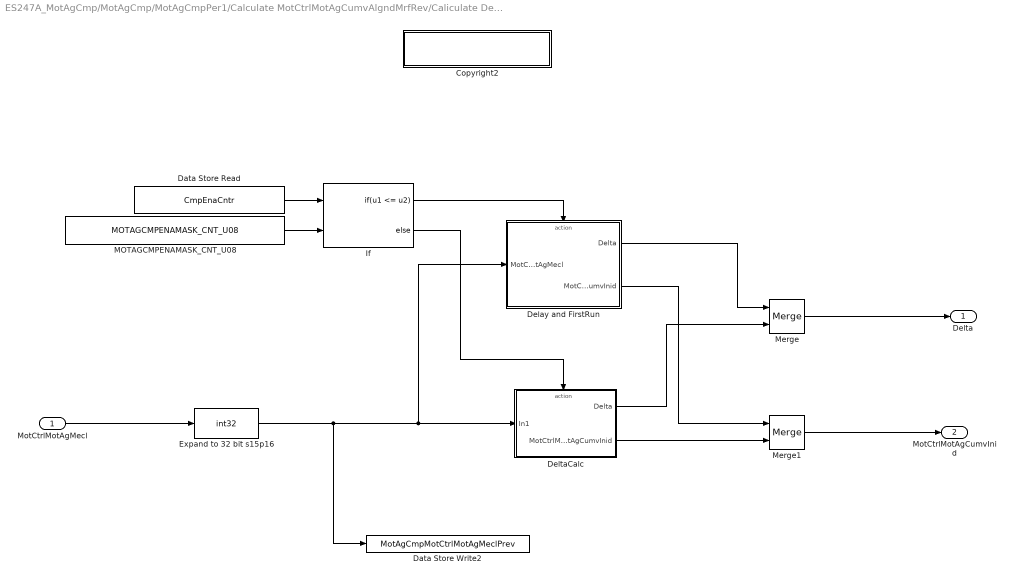
== system ES247A_MotAgCmp/MotAgCmp/MotAgCmpPer1/Calculate MotCtrlMotAgCumvAlgndMrfRev/Caliculate Delta ==
  MotCtrlMotAgMecl : Inport
  Copyright2 : Subsystem  Description=|  mask(Copyright Information){none=on}
      | Copyright info block.                                               
      |                                                                     
      | Place copyright information at the top of every subsystem in design.
      mask prompts: none "No parameters"
      mask help: Place copyright information at the top of every subsystem in design.
      mask Display:
      | NxtrConf = 'Nexteer Confidential';
      | 
      | sys = bdroot; %handle for the current model ("system")
      | first = get_param(sys,'Created');
      | if(isempty(first))
      |     first = datestr(now,'yyyy');
      | else
      |     first = first(end-3:end);  %year is last four digits
      | end
      | 
      | last = get_param(sys,'LastModifiedDate');
      | if isempty(last)
      |     last = datestr(now,'yyyy');
      | else
      |     last = last(end-3:end);
      | end
      | 
      | if strcmp(first,last)
      |     fprintf('%s\nCopyright  %s Nexteer',NxtrConf,first);
      | else
      |     fprintf('%s\n%s%s-%s Nexteer',NxtrConf,char(169),first,last);
      | end
  Data Store Read : DataStoreRead  DataStoreName=CmpEnaCntr
  Data Store Write2 : DataStoreWrite  Priority=2  DataStoreName=MotAgCmpMotCtrlMotAgMeclPrev
      settings: AttributesFormatString=Priority:%<Priority>
  Delay and FirstRun : Subsystem  Priority=1  TreatAsAtomicUnit=on
      settings: AttributesFormatString=Priority:%<Priority>
  DeltaCalc : Subsystem  Priority=1  TreatAsAtomicUnit=on
      settings: AttributesFormatString=Priority:%<Priority>
  Expand to 32 bit s15p16 : DataTypeConversion  RequirementInfo={} %GIDa_1c00d84a_0050_4ed2_a4a5_b1c46bcbc420  OutDataTypeStr=int32
  If : If  RequirementInfo={'linktype_rmi_doors' '0000cf60 (/E-STEER Core/SubSystem Specifications/Electrical Actuator/Control Module/FDD Module Requirements/EA4/ES247A_MotAgCmp)' '#ES247A_86' 'true' 'REQ: ES247A_86' '' } %GIDa_bfca5ed4_63b4_4fdf_8f63_c0ab4f9eca09  Priority=0  NumInputs=2  IfExpression=u1 <= u2
  MOTAGCMPENAMASK_CNT_U08 : Constant  RequirementInfo={'linktype_rmi_doors' '0000cf60 (/E-STEER Core/SubSystem Specifications/Electrical Actuator/Control Module/FDD Module Requirements/EA4/ES247A_MotAgCmp)' '#ES247A_86' 'true' 'REQ: ES247A_86' '' } %GIDa_13296f7c_2eb6_4f41_8946_017aa494cd9a  Value=MOTAGCMPENAMASK_CNT_U08
  Merge : Merge
  Merge1 : Merge
  Delta : Outport
  MotCtrlMotAgCumvInid : Outport  Port=2
  wires:
  MotCtrlMotAgMecl/1 -> Expand to 32 bit s15p16/1
  Expand to 32 bit s15p16/1 -> Data Store Write2/1, Delay and FirstRun/1(MotCtrlMotAgMecl), DeltaCalc/1(In1)
  Data Store Read/1 -> If/1
  Delay and FirstRun/1(Delta) -> Merge/1
  If/1 -> Delay and FirstRun/Action
  If/2 -> DeltaCalc/Action
  DeltaCalc/1(Delta) -> Merge/2
  Merge/1 -> Delta/1
  MOTAGCMPENAMASK_CNT_U08/1 -> If/2
  Delay and FirstRun/2(MotCtrlMotAgCumvInid) -> Merge1/1
  DeltaCalc/2(MotCtrlMotAgCumvInid) -> Merge1/2
  Merge1/1 -> MotCtrlMotAgCumvInid/1

== system ES247A_MotAgCmp/MotAgCmp/MotAgCmpPer1/Calculate MotCtrlMotAgCumvAlgndMrfRev/Copyright2 ==

== system ES247A_MotAgCmp/MotAgCmp/MotAgCmpPer1/Calculate MotCtrlMotAgCumvAlgndMrfRev/Caliculate Delta/Copyright2 ==

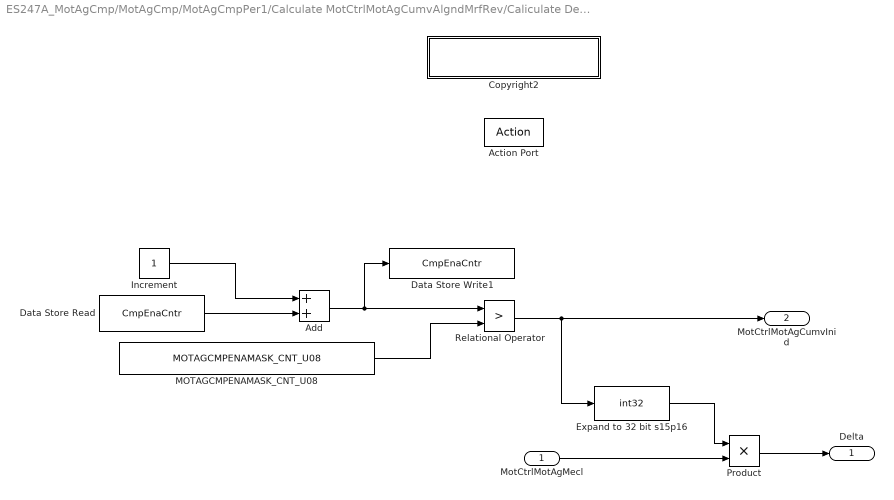
== system ES247A_MotAgCmp/MotAgCmp/MotAgCmpPer1/Calculate MotCtrlMotAgCumvAlgndMrfRev/Caliculate Delta/Delay and FirstRun ==
  MotCtrlMotAgMecl : Inport
  Action Port : ActionPort  ActionType=then
  Add : Sum
  Copyright2 : Subsystem  Description=|  mask(Copyright Information){none=on}
      | Copyright info block.                                               
      |                                                                     
      | Place copyright information at the top of every subsystem in design.
      mask prompts: none "No parameters"
      mask help: Place copyright information at the top of every subsystem in design.
      mask Display:
      | NxtrConf = 'Nexteer Confidential';
      | 
      | sys = bdroot; %handle for the current model ("system")
      | first = get_param(sys,'Created');
      | if(isempty(first))
      |     first = datestr(now,'yyyy');
      | else
      |     first = first(end-3:end);  %year is last four digits
      | end
      | 
      | last = get_param(sys,'LastModifiedDate');
      | if isempty(last)
      |     last = datestr(now,'yyyy');
      | else
      |     last = last(end-3:end);
      | end
      | 
      | if strcmp(first,last)
      |     fprintf('%s\nCopyright  %s Nexteer',NxtrConf,first);
      | else
      |     fprintf('%s\n%s%s-%s Nexteer',NxtrConf,char(169),first,last);
      | end
  Data Store Read : DataStoreRead  DataStoreName=CmpEnaCntr
  Data Store Write1 : DataStoreWrite  DataStoreName=CmpEnaCntr
  Expand to 32 bit s15p16 : DataTypeConversion  RequirementInfo={} %GIDa_8908a0b2_e512_49aa_9aac_68c3b59edb0d  OutDataTypeStr=int32
  Increment : Constant  OutDataTypeStr=uint8
  MOTAGCMPENAMASK_CNT_U08 : Constant  RequirementInfo={} %GIDa_5a9895f1_d24d_4e3f_a285_a77fec619921  Value=MOTAGCMPENAMASK_CNT_U08
  Product : Product  OutDataTypeStr=Inherit: Same as first input
  Relational Operator : RelationalOperator  Operator=>  OutDataTypeStr=boolean
  Delta : Outport
  MotCtrlMotAgCumvInid : Outport  Port=2
  wires:
  Increment/1 -> Add/1
  Data Store Read/1 -> Add/2
  MOTAGCMPENAMASK_CNT_U08/1 -> Relational Operator/2
  MotCtrlMotAgMecl/1 -> Product/2
  Product/1 -> Delta/1
  Relational Operator/1 -> MotCtrlMotAgCumvInid/1, Expand to 32 bit s15p16/1
  Expand to 32 bit s15p16/1 -> Product/1
  Add/1 -> Relational Operator/1, Data Store Write1/1

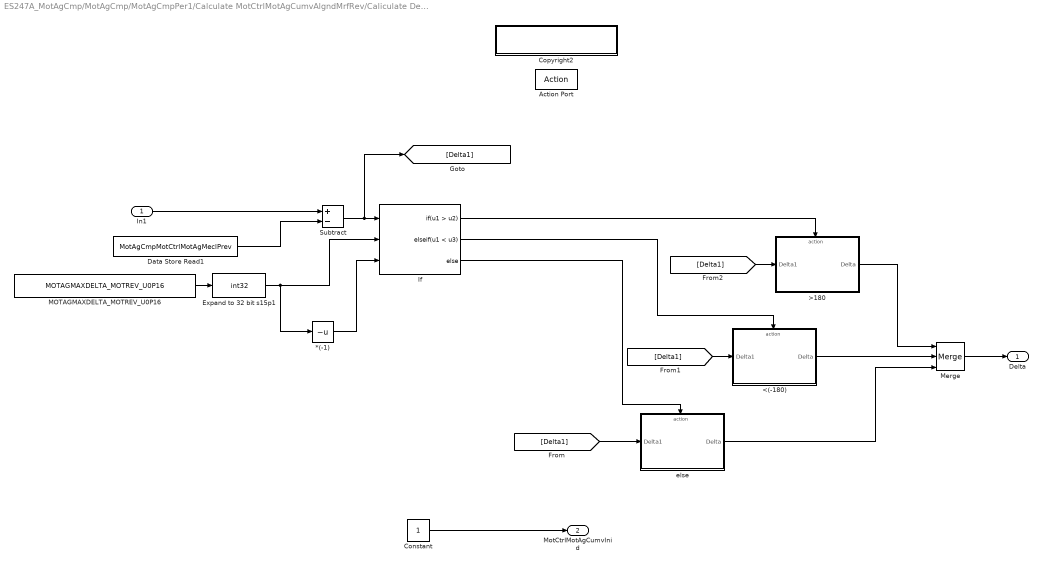
== system ES247A_MotAgCmp/MotAgCmp/MotAgCmpPer1/Calculate MotCtrlMotAgCumvAlgndMrfRev/Caliculate Delta/DeltaCalc ==
  In1 : Inport
  Action Port : ActionPort  ActionType=else
  *(-1) : UnaryMinus
  <(-180) : Subsystem  TreatAsAtomicUnit=on
  >180 : Subsystem  TreatAsAtomicUnit=on
  Constant : Constant  OutDataTypeStr=boolean
  Copyright2 : Subsystem  Description=|  mask(Copyright Information){none=on}
      | Copyright info block.                                               
      |                                                                     
      | Place copyright information at the top of every subsystem in design.
      mask prompts: none "No parameters"
      mask help: Place copyright information at the top of every subsystem in design.
      mask Display:
      | NxtrConf = 'Nexteer Confidential';
      | 
      | sys = bdroot; %handle for the current model ("system")
      | first = get_param(sys,'Created');
      | if(isempty(first))
      |     first = datestr(now,'yyyy');
      | else
      |     first = first(end-3:end);  %year is last four digits
      | end
      | 
      | last = get_param(sys,'LastModifiedDate');
      | if isempty(last)
      |     last = datestr(now,'yyyy');
      | else
      |     last = last(end-3:end);
      | end
      | 
      | if strcmp(first,last)
      |     fprintf('%s\nCopyright  %s Nexteer',NxtrConf,first);
      | else
      |     fprintf('%s\n%s%s-%s Nexteer',NxtrConf,char(169),first,last);
      | end
  Data Store Read1 : DataStoreRead  DataStoreName=MotAgCmpMotCtrlMotAgMeclPrev
  Expand to 32 bit s15p1 : DataTypeConversion  RequirementInfo={} %GIDa_64fed2c4_70c8_417d_a3be_c99224035913  OutDataTypeStr=int32
  If : If  NumInputs=3  IfExpression=u1 > u2  ElseIfExpressions=u1 < u3
  MOTAGMAXDELTA_MOTREV_U0P16 : Constant  RequirementInfo={'linktype_rmi_doors' '0000cf60 (/E-STEER Core/SubSystem Specifications/Electrical Actuator/Control Module/FDD Module Requirements/EA4/ES247A_MotAgCmp DRAFT)' '#ES247A_83' 'true' 'REQ: ES247A_83' '' } %GIDa_fade2d5b_4975_4926_8617_9e2b5c1ba556  Value=MOTAGMAXDELTA_MOTREV_U0P16
  Merge : Merge  Inputs=3
  Subtract : Sum  RequirementInfo={'linktype_rmi_doors' '0000cf60 (/E-STEER Core/SubSystem Specifications/Electrical Actuator/Control Module/FDD Module Requirements/EA4/ES247A_MotAgCmp)' '#ES247A_69' 'true' 'REQ: ES247A_69' '' } %GIDa_916431b0_f85f_46c9_84ce_edf75e2e1fa1  Inputs=+-
  else : Subsystem  TreatAsAtomicUnit=on
  Delta : Outport
  MotCtrlMotAgCumvInid : Outport  RequirementInfo={} %GIDa_294e6e86_b8b9_43cb_8d77_972091dfd069  Port=2
  wires:
  In1/1 -> Subtract/1
  MOTAGMAXDELTA_MOTREV_U0P16/1 -> Expand to 32 bit s15p1/1
  *(-1)/1 -> If/3
  If/1 -> >180/Action
  If/2 -> <(-180)/Action
  If/3 -> else/Action
  Subtract/1 -> [Delta1], If/1
  [Delta1] -> else/1(Delta1)
  [Delta1] -> <(-180)/1(Delta1)
  [Delta1] -> >180/1(Delta1)
  Expand to 32 bit s15p1/1 -> *(-1)/1, If/2
  Merge/1 -> Delta/1
  else/1(Delta) -> Merge/3
  <(-180)/1(Delta) -> Merge/2
  >180/1(Delta) -> Merge/1
  Constant/1 -> MotCtrlMotAgCumvInid/1
  Data Store Read1/1 -> Subtract/2

== system ES247A_MotAgCmp/MotAgCmp/MotAgCmpPer1/Calculate MotCtrlMotAgCumvAlgndMrfRev/Caliculate Delta/Delay and FirstRun/Copyright2 ==

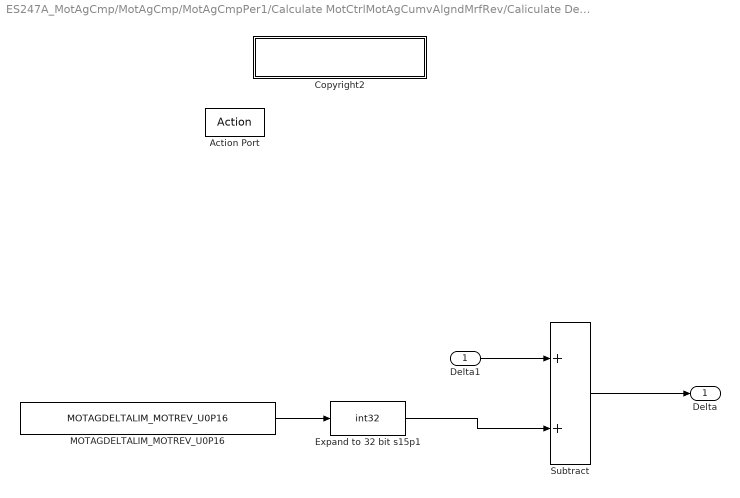
== system ES247A_MotAgCmp/MotAgCmp/MotAgCmpPer1/Calculate MotCtrlMotAgCumvAlgndMrfRev/Caliculate Delta/DeltaCalc/<(-180) ==
  Delta1 : Inport
  Action Port : ActionPort  ActionType=elseif
  Copyright2 : Subsystem  Description=|  mask(Copyright Information){none=on}
      | Copyright info block.                                               
      |                                                                     
      | Place copyright information at the top of every subsystem in design.
      mask prompts: none "No parameters"
      mask help: Place copyright information at the top of every subsystem in design.
      mask Display:
      | NxtrConf = 'Nexteer Confidential';
      | 
      | sys = bdroot; %handle for the current model ("system")
      | first = get_param(sys,'Created');
      | if(isempty(first))
      |     first = datestr(now,'yyyy');
      | else
      |     first = first(end-3:end);  %year is last four digits
      | end
      | 
      | last = get_param(sys,'LastModifiedDate');
      | if isempty(last)
      |     last = datestr(now,'yyyy');
      | else
      |     last = last(end-3:end);
      | end
      | 
      | if strcmp(first,last)
      |     fprintf('%s\nCopyright  %s Nexteer',NxtrConf,first);
      | else
      |     fprintf('%s\n%s%s-%s Nexteer',NxtrConf,char(169),first,last);
      | end
  Expand to 32 bit s15p1 : DataTypeConversion  RequirementInfo={} %GIDa_41f231b4_aac4_4b1c_b7ec_f41969dd47ae  OutDataTypeStr=int32
  MOTAGDELTALIM_MOTREV_U0P16 : Constant  RequirementInfo={} %GIDa_a1dd4bb1_7444_491e_85b7_8d4cad11aed5  Value=MOTAGDELTALIM_MOTREV_U0P16
  Subtract : Sum
  Delta : Outport
  wires:
  Delta1/1 -> Subtract/1
  MOTAGDELTALIM_MOTREV_U0P16/1 -> Expand to 32 bit s15p1/1
  Expand to 32 bit s15p1/1 -> Subtract/2
  Subtract/1 -> Delta/1
